simulink model "polydezim_4_"  (Simulink 7.8)
settings: Solver=FixedStepDiscrete  SolverMode=SingleTasking  StartTime=0.0  StopTime=10.0  RelTol=1e-3
values from neighbouring files (symbols this model uses):
  h = firpm(64,f,m)    [CFIR_1.m]    (also in adapt_filter1.m = adaptfilt.lms(ni,mu); adapt_filter2.m = adaptfilt.blms(ni,mu,1,36); adaptiv_2.m = [1 2 3 4 5 6 7 8 9 10]; adaptiv_3.m = [1 2 3 4 5 6 7 8 9 10])
  M = 2    [CFIR_1.m]    (also in block_lms_.m = 16; cic_dezim1.m = ',num2str(M),'; cic_dezim1_.m = ',num2str(M),     '; cic_dezim2.m = ',num2str(M),')
  Ts = 1/fs    (= 6.25e-05)    [G722_1.m]    (also in adaptiv_2.m = 0.001; adaptiv_3.m = 0.001; adaptiv_4.m = 0.001; adaptiv_5.m = 0.001)
undefined symbols (not defined in the file or in its folder): g, n_buffer
libraries: dspobslib x3, dspsigops x2
settings Model: Creator=svenhoffmann  LastModifiedBy=josef  ExtModeAutoUpdateStatusClock=off
settings DataIOCC: SignalLoggingName=sigsOut
settings OptimizationCC: InitFltsAndDblsToZero=on
settings DebuggingCC: SaveWithParameterizedLinksMsg=none  SignalResolutionControl=TryResolveAllWithWarning  SolverPrmCheckMsg=none  MultiTaskDSMMsg=warning  MultiTaskCondExecSysMsg=none  FcnCallInpInsideContextMsg=Use local settings  StrictBusMsg=None
settings HardwareCC: TargetUnknown=on
settings RTWCC: IncludeERTFirstTime=on
settings GRTTargetCC: TargetFcnLib=ansi_tfl_tmw.mat

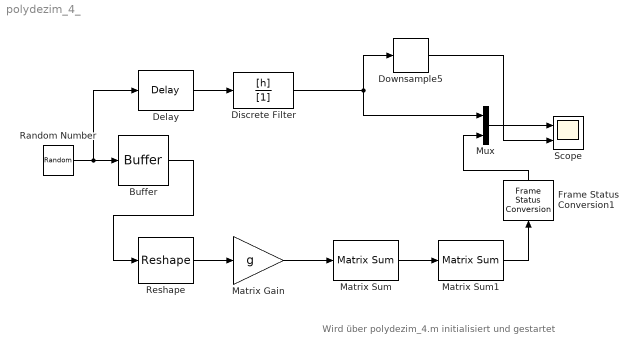
== system polydezim_4_ ==
  note: Wird über polydezim_4.m initialisiert und gestartet
  Buffer : Buffer  N=n_buffer  V=n_buffer-M
  Delay : dspsigops/Delay  InputProcessing=Inherited (this choice will be removed - see release notes)  dly_unit=Samples  delay=3  ic_detail=off  dif_ic_for_ch=off  dif_ic_for_dly=off  ic=0  reset_popup=None
  Discrete Filter : DiscreteFilter  Numerator=[h]  Denominator=[1]  SampleTime=Ts
  Downsample5 : dspsigops/Downsample  N=5  phase=0  InputProcessing=Inherited (this choice will be removed - see release notes)  RateOptions=Enforce single-rate processing  smode=Allow multirate  fmode=Maintain input frame size  ic=0
  Frame Status Conversion1 : dspobslib/Frame Status Conversion  growRefPort=off  outframe=Sample-based
  Matrix Gain : Gain  Gain=g  SaturateOnIntegerOverflow=on  OutDataTypeStr=Inherit: Same as input  ParamDataTypeStr=Inherit: Same as input
  Matrix Sum : dspobslib/Matrix Sum  Dim=Rows  roundingMode=Floor  overflowMode=off
  Matrix Sum1 : dspobslib/Matrix Sum  Dim=Columns  roundingMode=Floor  overflowMode=off
  Mux : Mux  Inputs=2
  Random Number : RandomNumber  SampleTime=Ts
  Reshape : Reshape  OutputDimensionality=Customize  OutputDimensions=[5,26]
  Scope : Scope  NumInputPorts=2
      settings: YMin=-5~-5  YMax=5~5
  wires:
  Discrete Filter/1 -> Mux/1, Downsample5/1
  Mux/1 -> Scope/1
  Random Number/1 -> Buffer/1, Delay/1
  Buffer/1 -> Reshape/1
  Downsample5/1 -> Scope/2
  Matrix Gain/1 -> Matrix Sum/1
  Matrix Sum/1 -> Matrix Sum1/1
  Matrix Sum1/1 -> Frame Status Conversion1/1
  Frame Status Conversion1/1 -> Mux/2
  Delay/1 -> Discrete Filter/1
  Reshape/1 -> Matrix Gain/1
